simulink model "BlueROV2_Exp_Simu"  (R2023b)
settings: Solver=FixedStepAuto  StartTime=0.0  StopTime=120  FixedStep=dt  RelTol=1e-3
values from neighbouring files (symbols this model uses):
  Af = diag(ti)    [RM_param_AGF.m]
  B = [zeros(6,6) ... (first row only)    [EKF_param.m]
  Ballast_Force = Ballast_Compute(Ballast_Config)    [Integrate.m]    (also in init.m = Ballast_Term(Ballast_Config); init_NIF.m = [0; 0; 0; 0; 0; 0]; init_NIF2.m = [0; 0; Ballast_Term; 0]; init_ODE.m)
  dt = 0.1    [Integrate.m]    (also in init.m; init_NIF.m; init_NIF2.m; init_ODE.m)
  Gamma = diag(omega_is)    [RM_param_AGF.m]
  Gamma_o = dt*E    [EKF_param.m]
  H = [eye(6), zeros(6,6) zeros(6,6)]    [EKF_param.m]
  inv_M = inv(Param.MT)    [EKF_param.m]
  inv_Tb = inv(Tb)    [EKF_param.m]
  Kd = [155; 355; 8985; 1205; 1205; 1]    [Integrate.m]    (also in init.m = [1; 1; 1; 1; 1; 1]; init_NIF.m; init_NIF2.m; init_ODE.m)
  Ki = [45; 45; 10; 96; 96; 1]    [Integrate.m]    (also in init.m = [1; 1; 1; 1; 1; 1]; init_NIF.m; init_NIF2.m; init_ODE.m)
  Kp = [255; 545; 7095; 2420; 2375; 1]    [Integrate.m]    (also in init.m = [1; 1; 1; 1; 1; 1]; init_NIF.m; init_NIF2.m; init_ODE.m)
  lower_limit = -upper_limit    (= -30)    [Integrate.m]    (also in init.m; init_NIF.m; init_NIF2.m; init_ODE.m)
  Omega = diag(2*omega_is.*zeta_is)    [RM_param_AGF.m]
  Param = BlueROV2_param()    [Integrate.m]    (also in init.m; init_NIF.m; init_NIF2.m; init_ODE.m)
  Q = diag([0.1,0.1,pi/180,1e6,1e6,1e9])*10e3    [EKF_param.m]
  R = diag([0.00001,0.00001,0.00001,      0.01*pi/180,0.01*pi/180,0.01*pi/180])*10e-4    [EKF_param.m]
  T_alloc = Thrust_Allocation()    [Integrate.m]    (also in init_NIF.m; init_NIF2.m; init_ODE.m; init_ballast_checking.m)
  T_alloc_ps = pinv(T_alloc' * T_alloc + lambda * eye(size(T_alloc, 2))) * T_alloc'    [Integrate.m]    (also in init_NIF.m; init_NIF2.m; init_ODE.m; init_ballast_checking.m)
  Tether_Force = zeros(6,1)    [Integrate.m]    (also in init.m; init_NIF.m; init_NIF2.m; init_ODE.m)
  thrust_rate = 5    [Integrate.m]    (also in init.m; init_NIF.m; init_NIF2.m; init_ODE.m)
  upper_limit = 30    [Integrate.m]    (also in init.m; init_NIF.m; init_NIF2.m; init_ODE.m)
undefined symbols (not defined in the file or in its folder): model_val, Phi_ref, Psi_ref, Theta_ref, time_stamps_phi, time_stamps_psi, time_stamps_theta, time_stamps_x, time_stamps_y, time_stamps_z, time_val, X_ref, Y_ref, Z_ref
libraries: slpidlib x6
(part 2 of 2)

== matlab function BlueROV2_Exp_Simu/Controller (PID)/To use/Rotation Matrix ==
  data: phi input; J_Theta_trp output; theta input; psi input
function J_Theta_trp  = Jacobian(phi, theta, psi)
%%%%%%%%%%%%%%%%%%%%%%%%%%%%%%%%%%%%%%%%%%%%%%%%%%%%%%%%%%%%%%%%%%%%%%%%%%%
% Command                                                                 %
%                                                                         %              
% Compute the Jacobian to integrate the next acceleration to velocity     %
%                                                                         %
% For 6-DOF Equations:                                                    %
% [ndot = Jacobian(n_theta) * v]                                          %
% -ndot = velocity expressed in NED frame                                 %
% -n_theta = rotational part of position vector                           %
% - v = velocity expressed in Body frame                                  %
%                                                                         %
% Argument:                                                               %
% X     : Input positional vector                                         %
%                                                                         %
% Created:      27.09.2023	Andreas Sitorus                               %
%                                                                         %
%%%%%%%%%%%%%%%%%%%%%%%%%%%%%%%%%%%%%%%%%%%%%%%%%%%%%%%%%%%%%%%%%%%%%%%%%%%
%% Linear Velocity Transformation Matrix
% Element
r11 = cos(psi) * cos(theta);
r12 = -sin(psi) * cos(phi) + cos(psi) * sin(theta) * sin(phi);
r13 = sin(psi) * sin(phi) + cos(psi) * cos(phi) * sin(theta);
r21 = sin(psi) * cos(theta);
r22 = cos(psi) * cos(phi) + sin(phi) * sin(theta) * sin(psi);
r23 = -cos(psi) * sin(phi) + sin(theta) * sin(psi) * cos(phi);
r31 = -sin(theta);
r32 = cos(theta) * sin(phi);
r33 = cos(theta) * cos(phi);

% Matrix
R_Theta = [r11 r12 r13;
           r21 r22 r23;
           r31 r32 r33];

%% Angular Velocity Transformation Matrix
% Element
t11 = 1;
t12 = sin(phi) * tan(theta);
t13 = cos(phi) * tan(theta);
t21 = 0;
t22 = cos(phi);
t23 = -sin(phi);
t31 = 0;
t32 = sin(phi) / cos(theta);
t33 = cos(phi) / cos(theta);

% Matrix
T_Theta = [t11 t12 t13;
           t21 t22 t23;
           t31 t32 t33];

%% Jacobian
J_Theta = [R_Theta  zeros(3);
           zeros(3) T_Theta];
J_Theta_trp = J_Theta';

end

== matlab function BlueROV2_Exp_Simu/Controller (PID)/To use/Rotation Matrix1 ==
  data: phi input; J_Theta_trp output; theta input; psi input
function J_Theta_trp  = Jacobian(phi, theta, psi)
%%%%%%%%%%%%%%%%%%%%%%%%%%%%%%%%%%%%%%%%%%%%%%%%%%%%%%%%%%%%%%%%%%%%%%%%%%%
% Command                                                                 %
%                                                                         %              
% Compute the Jacobian to integrate the next acceleration to velocity     %
%                                                                         %
% For 6-DOF Equations:                                                    %
% [ndot = Jacobian(n_theta) * v]                                          %
% -ndot = velocity expressed in NED frame                                 %
% -n_theta = rotational part of position vector                           %
% - v = velocity expressed in Body frame                                  %
%                                                                         %
% Argument:                                                               %
% X     : Input positional vector                                         %
%                                                                         %
% Created:      27.09.2023	Andreas Sitorus                               %
%                                                                         %
%%%%%%%%%%%%%%%%%%%%%%%%%%%%%%%%%%%%%%%%%%%%%%%%%%%%%%%%%%%%%%%%%%%%%%%%%%%
%% Linear Velocity Transformation Matrix
% Element
r11 = cos(psi) * cos(theta);
r12 = -sin(psi) * cos(phi) + cos(psi) * sin(theta) * sin(phi);
r13 = sin(psi) * sin(phi) + cos(psi) * cos(phi) * sin(theta);
r21 = sin(psi) * cos(theta);
r22 = cos(psi) * cos(phi) + sin(phi) * sin(theta) * sin(psi);
r23 = -cos(psi) * sin(phi) + sin(theta) * sin(psi) * cos(phi);
r31 = -sin(theta);
r32 = cos(theta) * sin(phi);
r33 = cos(theta) * cos(phi);

% Matrix
R_Theta = [r11 r12 r13;
           r21 r22 r23;
           r31 r32 r33];

%% Angular Velocity Transformation Matrix
% Element
t11 = 1;
t12 = sin(phi) * tan(theta);
t13 = cos(phi) * tan(theta);
t21 = 0;
t22 = cos(phi);
t23 = -sin(phi);
t31 = 0;
t32 = sin(phi) / cos(theta);
t33 = cos(phi) / cos(theta);

% Matrix
T_Theta = [t11 t12 t13;
           t21 t22 t23;
           t31 t32 t33];

%% Jacobian
J_Theta = [R_Theta  zeros(3);
           zeros(3) T_Theta];
J_Theta_trp = J_Theta';

end

== matlab function BlueROV2_Exp_Simu/Observer (EKF)/MATLAB Function ==
  data: y input; P_update output; U input; P input; states input; inv_M input; B input; H input; R input; Q input; dt input; inv_Tb input; Gamma_o input; states_update output; states_hat output; error output; K output
function [P_update, states_update, states_hat, error, K] = EKF(y, U, P, states, inv_M, B, H, R, Q, dt, inv_Tb, Gamma_o)
global Param
%% Update Parameters
% States
eta = states(1:6,:);
b = states(7:12,:);
nu = states(13:18,:);

% Position
x = eta(1);
y = eta(2);
z = eta(3);
phi = eta(4);
theta = eta(5);
psi = eta(6);

% Velocity
u = nu(1);
v = nu(2);
w = nu(3);
p = nu(4);
q = nu(5);
r = nu(6);

%% Compute f(x) + Bu
% Linear Velocity Transformation Matrix
% Element
r11 = cos(psi) * cos(theta);
r12 = -sin(psi) * cos(phi) + cos(psi) * sin(theta) * sin(phi);
r13 = sin(psi) * sin(phi) + cos(psi) * cos(phi) * sin(theta);
r21 = sin(psi) * cos(theta);
r22 = cos(psi) * cos(phi) + sin(phi) * sin(theta) * sin(psi);
r23 = -cos(psi) * sin(phi) + sin(theta) * sin(psi) * cos(phi);
r31 = -sin(theta);
r32 = cos(theta) * sin(phi);
r33 = cos(theta) * cos(phi);

% Matrix
R_Theta = [r11 r12 r13;
           r21 r22 r23;
           r31 r32 r33];

% Angular Velocity Transformation Matrix
% Element
t11 = 1;
t12 = sin(phi) * tan(theta);
t13 = cos(phi) * tan(theta);
t21 = 0;
t22 = cos(phi);
t23 = -sin(phi);
t31 = 0;
t32 = sin(phi) / cos(theta);
t33 = cos(phi) / cos(theta);

% Matrix
T_Theta = [t11 t12 t13;
           t21 t22 t23;
           t31 t32 t33];

% Rotation Matrix
Rot = [R_Theta  zeros(3);
       zeros(3) T_Theta];

fx = [Rot*nu;
      -inv_Tb*b;
      -inv_M*(Param.Fc_o + Param.Fd_o + Param.Fr_o + Param.g0 + rot_tot'*b)];

F = (B*U) + fx;

%% Predictor
% Linearization with Taylor Series Expansion
A = [zeros(6,12) rot_tot;
     zeros(6,6) -inv_Tb zeros(6,6)
     zeros(6,12) inv_M];

Phi = eye(18) + dt*A;

% Compute Estimated Error Covariance Propagation
P_hat = Phi*P*Phi' + Gamma_o*Q*Gamma_o';

% Compute Estimated States Propagation
states_hat = states + dt*F;


%% Corrector
% Kalman Gain
K = P_hat*H'/(H*P_hat*H'+R);

% Compute Estimated Error Covariance Update
P_update = (eye(15)-K*H)*P_hat*(eye(15)-K*H)' + K*R*K';

% Compute Estimated States Update
states_update = states_hat + K*(y-H*states_hat);

% Compute Error
error = y - H*states_hat;
end

== matlab function BlueROV2_Exp_Simu/Observer (EKF)/MATLAB Function1 ==
  data: states_vector input; eta_hat output; nu_hat output
function [eta_hat, nu_hat] = split_states(states_vector)
%%states [zeta,eta, b, nu] --15x1
%zeta - 6x1, 
%eta - 3x1, 
%b - 3x1, 
%nu - 3x1
eta_hat = states_vector(7:9,1);
nu_hat = states_vector(13:15,1);

end

== matlab function BlueROV2_Exp_Simu/Controller (PID)/Transformation_bn Position ==
  data: eta_n input; J_Theta_bn output
function J_Theta_bn  = Transform_bn(eta_n)
%%%%%%%%%%%%%%%%%%%%%%%%%%%%%%%%%%%%%%%%%%%%%%%%%%%%%%%%%%%%%%%%%%%%%%%%%%%
% Command                                                                 %
%                                                                         %
% Compute the Jacobian from {b} to {n}                                    %
%                                                                         %
% For 6-DOF Equations:                                                    %
% [ndot = Jacobian(n_theta) * v]                                          %
% -ndot = velocity expressed in NED frame                                 %
% -n_theta = rotational part of position vector                           %
% - v = velocity expressed in Body frame                                  %
%                                                                         %
% Argument:                                                               %
% eta     : Input positional vector                                       %
%                                                                         %
% Created:      27.09.2023	Andreas Sitorus                               %
%                                                                         %
%%%%%%%%%%%%%%%%%%%%%%%%%%%%%%%%%%%%%%%%%%%%%%%%%%%%%%%%%%%%%%%%%%%%%%%%%%%
%% Get the angular velocity
phi = eta_n(4);       % Rolling angle
theta = eta_n(5);     % Pitching angle
psi = eta_n(6);       % Yaw angle

%% Linear Velocity Transformation Matrix
% Element
r11 = cos(psi) * cos(theta);
r12 = -sin(psi) * cos(phi) + cos(psi) * sin(theta) * sin(phi);
r13 = sin(psi) * sin(phi) + cos(psi) * cos(phi) * sin(theta);
r21 = sin(psi) * cos(theta);
r22 = cos(psi) * cos(phi) + sin(phi) * sin(theta) * sin(psi);
r23 = -cos(psi) * sin(phi) + sin(theta) * sin(psi) * cos(phi);
r31 = -sin(theta);
r32 = cos(theta) * sin(phi);
r33 = cos(theta) * cos(phi);

% Rotation Matrix (from {b} to {n})
R_Theta_nb = [r11 r12 r13;
              r21 r22 r23;
              r31 r32 r33];

%% Angular Velocity Transformation Matrix
% Element
t11 = 1;
t12 = sin(phi) * tan(theta);
t13 = cos(phi) * tan(theta);
t21 = 0;
t22 = cos(phi);
t23 = -sin(phi);
t31 = 0;
t32 = sin(phi) / cos(theta);
t33 = cos(phi) / cos(theta);

% Angular Velocity Rotation Matrix (from {b} to {n})
T_Theta_nb = [t11 t12 t13;
              t21 t22 t23;
              t31 t32 t33];

%% Jacobian
J_Theta_nb = [R_Theta_nb  zeros(3);
              zeros(3) T_Theta_nb];
J_Theta_bn = J_Theta_nb';
end
